simulink model "motor_sim"  (R2026a)
settings: Solver=VariableStepAuto
settings Model: Creator=codykremer  LastModifiedBy=codykremer

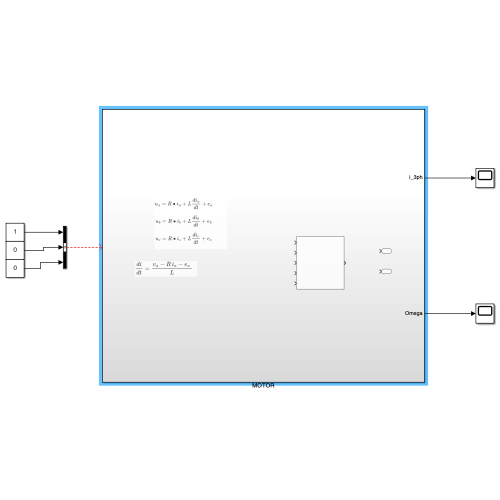
[thumbnail: Simulink's stored preview of the top-level diagram]
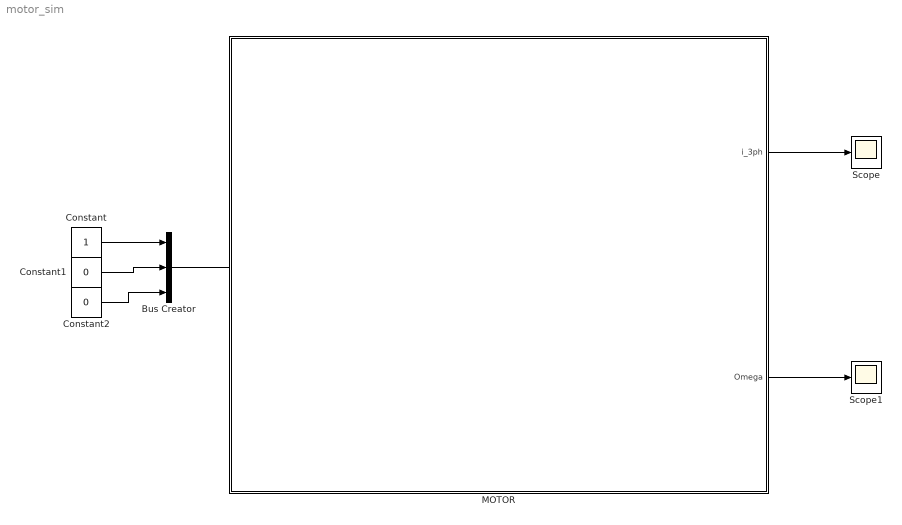
== system motor_sim ==
  Bus Creator : BusCreator  Inputs=3
  Constant : Constant
  Constant1 : Constant  Value=0
  Constant2 : Constant  Value=0
  MOTOR : Subsystem
  Scope : Scope
      settings: ActiveDisplayYMinimum=-35.374985400665508  ActiveDisplayYMaximum=22.917130577261844
  Scope1 : Scope
  wires:
  MOTOR/1(i_3ph) -> Scope/1
  MOTOR/2(Omega) -> Scope1/1
  Bus Creator/1 -> ?
  Constant/1 -> Bus Creator/1
  Constant1/1 -> Bus Creator/2
  Constant2/1 -> Bus Creator/3

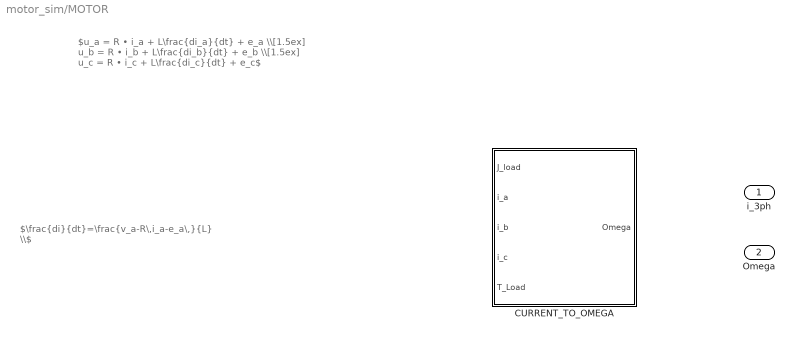
== system motor_sim/MOTOR ==
  note: $\frac{di}{dt}=\frac{v_a-R\,i_a-e_a\,}{L} \\$
  note: $u_a = R • i_a + L\frac{di_a}{dt} + e_a \\[1.5ex] u_b = R • i_b + L\frac{di_b}{dt} + e_b \\[1.5ex] u_c = R • i_c + L\frac{di_c}{dt} + e_c$
  CURRENT_TO_OMEGA : Subsystem
  i_3ph : Outport
  Omega : Outport  Port=2

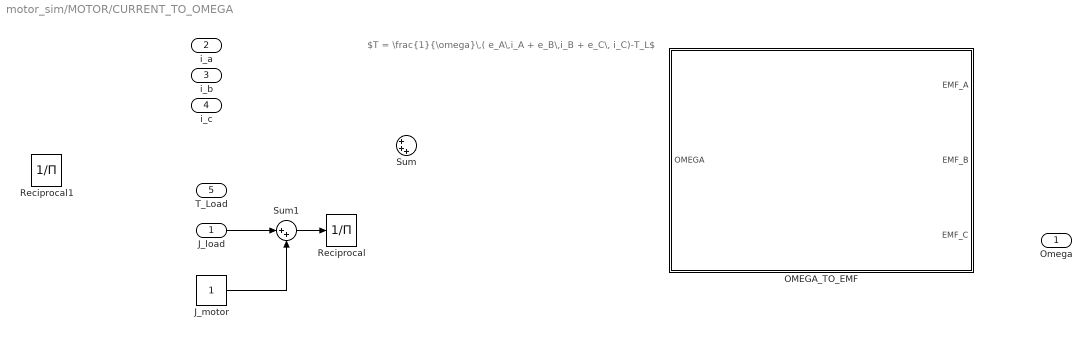
== system motor_sim/MOTOR/CURRENT_TO_OMEGA ==
  note: $T = \frac{1}{\omega}\,( e_A\,i_A + e_B\,i_B + e_C\, i_C)-T_L$
  J_load : Inport
  i_a : Inport  Port=2
  i_b : Inport  Port=3
  i_c : Inport  Port=4
  T_Load : Inport  Port=5
  J_motor : Constant
  OMEGA_TO_EMF : Subsystem
  Reciprocal : Product  Inputs=/
  Reciprocal1 : Product  Inputs=/
  Sum : Sum  Inputs=|+++
  Sum1 : Sum  Inputs=|++
  Omega : Outport
  wires:
  ? -> Omega/1
  Sum1/1 -> Reciprocal/1
  J_load/1 -> Sum1/1
  J_motor/1 -> Sum1/2

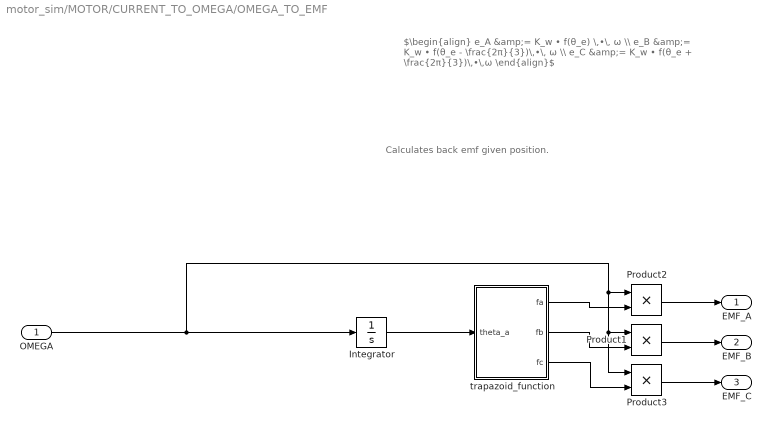
== system motor_sim/MOTOR/CURRENT_TO_OMEGA/OMEGA_TO_EMF ==
  note: Calculates back emf given position.
  note: $\begin{align} e_A &amp;= K_w • f(θ_e) \,•\, ω \\ e_B &amp;= K_w • f(θ_e - \frac{2π}{3})\,•\, ω \\ e_C &amp;= K_w • f(θ_e + \frac{2π}{3})\,•\,ω \end{align}$
  OMEGA : Inport
  Integrator : Integrator
  Product1 : Product
  Product2 : Product
  Product3 : Product
  trapazoid_function : MATLAB Function  TreatAsAtomicUnit=on
  EMF_A : Outport
  EMF_B : Outport  Port=2
  EMF_C : Outport  Port=3
  wires:
  Product2/1 -> EMF_A/1
  OMEGA/1 -> Integrator/1, Product3/1, Product1/1, Product2/1
  Integrator/1 -> trapazoid_function/1(theta_a)
  Product1/1 -> EMF_B/1
  Product3/1 -> EMF_C/1
  trapazoid_function/1(fa) -> Product2/2
  trapazoid_function/2(fb) -> Product1/2
  trapazoid_function/3(fc) -> Product3/2

== matlab function motor_sim/MOTOR/CURRENT_TO_OMEGA/OMEGA_TO_EMF/trapazoid_function ==
  data: theta_a input; fa output; fb output; fc output
function [fa, fb, fc]  = trapBEMF(theta_a)
    theta = mod(theta_a, 360);
    fa = shape(theta);
    fb = shape(mod(theta, 360));
    fc = shape(mod(theta - 240, 360));
end

function f = shape(t)
    if t < 120
        f = 1;
    elseif t < 180
        f = 1 - 2*(t-120)/60;
    elseif t < 300
        f = -1;
    else
        f = -1 + 2*(t-300)/60;
    end
end
